simulink model "PIhigh"  (R2025a)
settings: Solver=VariableStepAuto  StartTime=0.0  StopTime=0.05  MaxStep=1e-9  RelTol=1e-3
libraries: spsVoltageMeasurementLib x5, spsSeriesRLCBranchLib x4, spsCurrentMeasurementLib x4, spsDiodeLib x2, spsMosfetLib x2, spsDCVoltageSourceLib x1, spsLinearTransformerLib x1, sps_lib x1
settings Model: Creator=FCH  LastModifiedBy=FCH
settings DataIOCC: ReturnWorkspaceOutputs=off

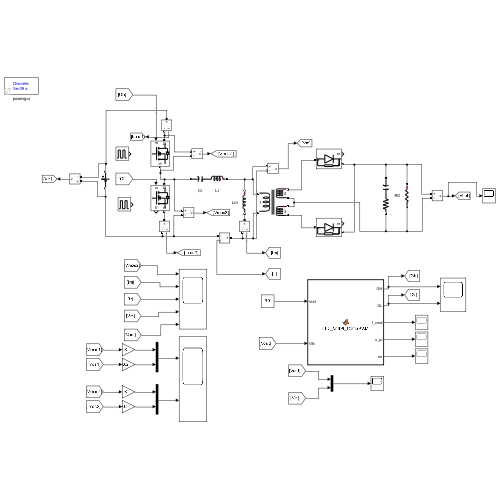
[thumbnail: Simulink's stored preview of the top-level diagram]
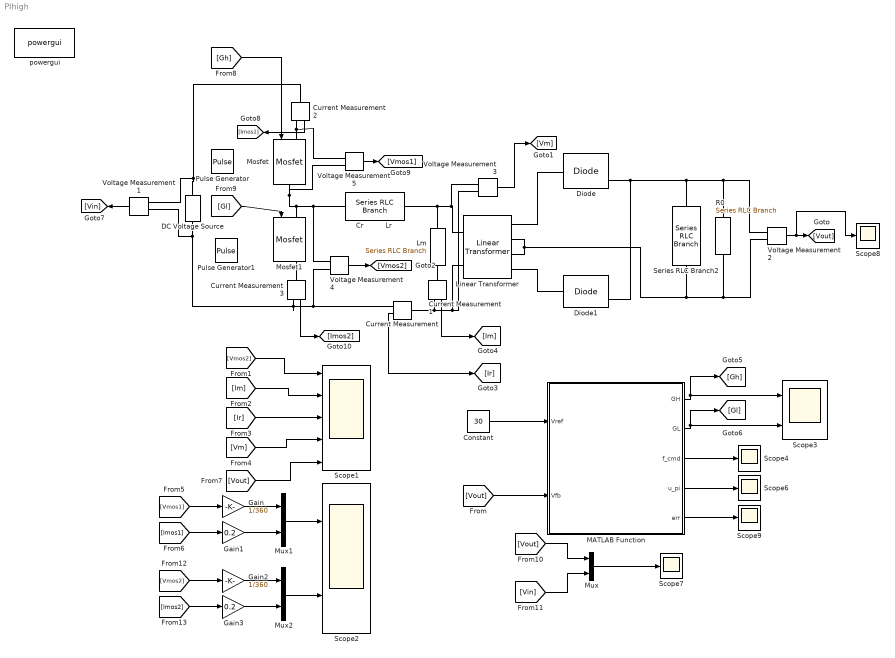
== system PIhigh ==
  Constant : Constant  Value=30
  Cr           Lr : spsSeriesRLCBranchLib/Series RLC Branch  LConnTagsString=__new0  RConnTagsString=__new0  BranchType=LC  Resistance=1  Inductance=18e-6  SetiL0=off  InitialCurrent=0  Capacitance=36e-9  Setx0=off  InitialVoltage=0  Measurements=None
  Current Measurement{,1..3} (4 alike) : spsCurrentMeasurementLib/Current Measurement  PhasorSimulation=off  OutputType=Complex  PSBequivalent=0
  DC Voltage Source : spsDCVoltageSourceLib/DC Voltage Source  Amplitude=400  Measurements=None
  Diode : spsDiodeLib/Diode  Ron=0.001  Lon=0  Vf=0.8  IC=0  UseSnubber=0  Rs=500  Cs=250e-9  Measurements=on
  Diode1 : spsDiodeLib/Diode  Ron=0.001  Lon=0  Vf=0.8  IC=0  UseSnubber=0  Rs=500  Cs=250e-9  Measurements=on
  Gain : Gain  Gain=1/360
  Gain1 : Gain  Gain=0.2
  Gain2 : Gain  Gain=1/360
  Gain3 : Gain  Gain=0.2
  Linear Transformer : spsLinearTransformerLib/Linear Transformer  UNITS=SI  NominalPower=[ 250e2 180e3 ]  winding1=[10 0 0]  winding2=[1 0 0]  ThreeWindings=on  winding3=[1 0 0]  RmLm=[inf inf]  Measurements=None  DataType=on
  Lm : spsSeriesRLCBranchLib/Series RLC Branch  LConnTagsString=__new0  RConnTagsString=__new0  BranchType=L  Resistance=1  Inductance=100e-6  SetiL0=off  InitialCurrent=0  Capacitance=1e-6  Setx0=off  InitialVoltage=0  Measurements=None
  MATLAB Function : MATLAB Function  TreatAsAtomicUnit=on
  Mosfet : spsMosfetLib/Mosfet  Ron=0.1  Lon=0  Rd=0.01  Vfd=0  IC=0  Rs=1e5  Cs=389e-1  Measurements=off
  Mosfet1 : spsMosfetLib/Mosfet  Ron=0.1  Lon=0  Rd=0.01  Vfd=0  IC=0  Rs=1e5  Cs=389e-12  Measurements=on
  Mux : Mux  Inputs=2
  Mux1 : Mux  Inputs=2
  Mux2 : Mux  Inputs=2
  Pulse Generator : DiscretePulseGenerator  PulseType=Time based  Period=1/270e2  PulseWidth=45
  Pulse Generator1 : DiscretePulseGenerator  PulseType=Time based  Period=1/270e2  PulseWidth=45  PhaseDelay=180/360*1/270e2
  R0 : spsSeriesRLCBranchLib/Series RLC Branch  LConnTagsString=__new0  RConnTagsString=__new0  BranchType=R  Resistance=10000  Inductance=1e-3  SetiL0=off  InitialCurrent=0  Capacitance=1e-6  Setx0=off  InitialVoltage=0  Measurements=Branch voltage
  Scope1 : Scope  NumInputPorts=5
      settings: ActiveDisplayYMinimum=-45.097156746790269  ActiveDisplayYMaximum=405.0968315999923
  Scope2 : Scope  NumInputPorts=2
      settings: ActiveDisplayYMinimum=-2.2545286858856493  ActiveDisplayYMaximum=1.9388480706148599
  Scope3 : Scope  NumInputPorts=2
      settings: ActiveDisplayYMinimum=-0.12499999999999997  ActiveDisplayYMaximum=1.125  DataLoggingVariableName=ScopeData3
  Scope{4,6..9} (5 alike) : Scope
      Scope4 settings: ActiveDisplayYMinimum=214374.4138129011  ActiveDisplayYMaximum=228140.57300499929  DataLoggingVariableName=ScopeData4
      Scope6 settings: ActiveDisplayYMinimum=-44.999999999999972  ActiveDisplayYMaximum=404.99999999999994  DataLoggingVariableName=ScopeData6
      Scope7 settings: ActiveDisplayYMinimum=-44.999999999999972  ActiveDisplayYMaximum=404.99999999999994  DataLoggingVariableName=ScopeData2
      Scope8 settings: ActiveDisplayYMinimum=-6.1893685032288337  ActiveDisplayYMaximum=55.704316529059234  DataLoggingVariableName=U_output
      Scope9 settings: ActiveDisplayYMinimum=-25.704316529059234  ActiveDisplayYMaximum=36.189368503228835  DataLoggingVariableName=ScopeData8
  Series RLC Branch2 : spsSeriesRLCBranchLib/Series RLC Branch  LConnTagsString=__new0  RConnTagsString=__new0  BranchType=RC  Resistance=0.01  Inductance=1e-3  SetiL0=off  InitialCurrent=0  Capacitance=1e-6  Setx0=off  InitialVoltage=0  Measurements=None
  Voltage Measurement{1..5} (5 alike) : spsVoltageMeasurementLib/Voltage Measurement  PhasorSimulation=off  OutputType=Complex  PSBequivalent=0
  powergui : sps_lib/powergui  Priority=1  SimulationMode=Discrete  SampleTime=1/(200e6)  frequency=60  Iterations=50  frequencyindice=0  Pbase=100e6  ErrMax=1e-4  UnitsV=kV  UnitsW=MW  buscounter=0  FunctionMessages=off  echomessages=off  EnableUseOfTLC=off  CurrentSourceSwitches=off  DisableSnubberDevices=off  DisableRonSwitches=off  DisableVfSwitches=off  DisplayEquations=off  AutomaticDiscreteSolvers=off  SolverType=Tustin/Backward Euler (TBE)  Interpol=off  ExternalGateDelay=off  methode=off  Ts=100  x0status=blocks  SPID=on  SwTol=0  HookPort=off  NonlinearTolerance=1e-4  nMaxIteration=100  ContinueOnMaxIteration=off  RestoreLinks=warning  ResistiveCurrentMeasurement=off  Frange=[0:2:500]  Ylog=off  Xlog=on  ShowGrid=off  save=off  variable=ZData  structure=0  ZoomFFT=off  StartTime=0.0  cycles=1  DisplayStyle=1  fundamental=60  FreqAxis=off  MaxFrequency=1000  frequencyindicesteady=1  RmsSteady=1  display=off
  wires:
  Voltage Measurement2/1 -> Scope8/1, [Vout]
  Constant/1 -> MATLAB Function/1(Vref)
  [Vout] -> MATLAB Function/2(Vfb)
  MATLAB Function/1(GH) -> [Gh], Scope3/1
  MATLAB Function/2(GL) -> [Gl], Scope3/2
  MATLAB Function/4(u_pi) -> Scope6/1
  MATLAB Function/3(f_cmd) -> Scope4/1
  MATLAB Function/5(err) -> Scope9/1
  Voltage Measurement3/1 -> [Vm]
  Voltage Measurement4/1 -> [Vmos2]
  Current Measurement/1 -> [Ir]
  Current Measurement1/1 -> [Im]
  [Vmos2] -> Scope1/1
  [Im] -> Scope1/2
  [Ir] -> Scope1/3
  [Vm] -> Scope1/4
  [Vout] -> Scope1/5
  Mux/1 -> Scope7/1
  [Vout] -> Mux/1
  Voltage Measurement1/1 -> [Vin]
  [Vin] -> Mux/2
  [Gl] -> Mosfet1/1
  [Gh] -> Mosfet/1
  Current Measurement2/1 -> [Imos1]
  Voltage Measurement5/1 -> [Vmos1]
  Current Measurement3/1 -> [Imos2]
  [Vmos1] -> Gain/1
  [Imos1] -> Gain1/1
  Mux1/1 -> Scope2/1
  [Vmos2] -> Gain2/1
  [Imos2] -> Gain3/1
  Mux2/1 -> Scope2/2
  Gain/1 -> Mux1/1
  Gain1/1 -> Mux1/2
  Gain2/1 -> Mux2/1
  Gain3/1 -> Mux2/2
  connections:
  DC Voltage Source/RConn1 -- Voltage Measurement1/LConn2 -- Current Measurement2/LConn1
  Mosfet/RConn1 -- Voltage Measurement4/LConn1 -- Cr           Lr/RConn1 -- Mosfet1/LConn1 -- Voltage Measurement5/LConn2
  Lm/RConn1 -- Current Measurement1/LConn1
  Cr           Lr/LConn1 -- Voltage Measurement3/LConn1 -- Linear Transformer/LConn1 -- Lm/LConn1
  Linear Transformer/RConn1 -- Diode/LConn1
  Diode/RConn1 -- Diode1/RConn1 -- Series RLC Branch2/RConn1 -- R0/LConn1 -- Voltage Measurement2/LConn1
  R0/RConn1 -- Voltage Measurement2/LConn2 -- Linear Transformer/RConn2 -- Linear Transformer/RConn3 -- Series RLC Branch2/LConn1
  Linear Transformer/RConn4 -- Diode1/LConn1
  Current Measurement/RConn1 -- Voltage Measurement1/LConn1 -- DC Voltage Source/LConn1 -- Current Measurement3/RConn1 -- Voltage Measurement4/LConn2
  Linear Transformer/LConn2 -- Voltage Measurement3/LConn2 -- Current Measurement1/RConn1 -- Current Measurement/LConn1
  Current Measurement2/RConn1 -- Voltage Measurement5/LConn1 -- Mosfet/LConn1
  Mosfet1/RConn1 -- Current Measurement3/LConn1

== matlab function PIhigh/MATLAB Function ==
  data: Vref input; GH output; Vfb input; GL output; f_cmd output; u_pi output; err output
 function [GH, GL, f_cmd, u_pi,err] = LLC_VoltPI_CompPWM(Vref, Vfb)
%#codegen
% LLC 变换器 PI 电压闭环 + 互补 PWM 驱动（变频控制）
% 输入:
%   Vref  - 输出电压给定 (V)
%   Vfb   - 输出电压反馈 (V)
% 输出:
%   GH    - 高桥臂驱动（逻辑 0/1）
%   GL    - 低桥臂驱动（逻辑 0/1），与 GH 互补且带死区
%   f_cmd - 当前开关频率命令 (Hz)，便于观察
%   u_pi  - PI 控制器输出（归一化调节量，便于调试）

%% ========= 用户根据实际系统需要修改的参数 =========

% --- 控制周期（与 MATLAB Function 调用步长一致） ---
% Ts = 1/(270e3*20);          % 1 us 控制周期，例如 MCU 1 MHz ISR
Ts = 1/(2000e6);          % 1 us 控制周期，例如 MCU 1 MHz ISR
% --- PI 参数（电压环）---
Kp = 0.00001;           % 比例系数
Ki = 50;            % 积分系数

% --- LLC 开关频率范围 ---
f_min = 180e3;       % 最低频率 (Hz)
f_max = 270e3;      % 最高频率 (Hz)

% --- 死区时间 ---
t_dead = 200e-9;    % 2 ns 死区，根据驱动/器件调整

% --- 积分项限幅，防止积分饱和 ---
ui_max = 0.5;
ui_min = -0.5;

%% ========= 持久变量（只初始化一次） =========
persistent ui t_half leg dead_t
if isempty(ui)
    ui      = 0;        % PI 积分项
    t_half  = 0;        % 半周期计时
    leg     = int8(0);  % 当前导通臂：0=上臂导通，1=下臂导通
    dead_t  = 0;        % 当前死区计时
end

%% ========= 1. 电压误差 & PI 电压环 =========
err = Vref - Vfb;      % 电压误差：Vref - Vfb

% 比例项
up = Kp * err;

% 积分项更新
ui = ui + Ki * Ts * err;

% 积分限幅
if ui > ui_max
    ui = ui_max;
elseif ui < ui_min
    ui = ui_min;
end

% PI 输出
u_pi = up + ui;

%% ========= 2. PI 输出映射为开关频率命令 =========
% 假设 u_pi 在 [-1, 1] 范围内有效，这里再做一次限幅
if u_pi > 1
    u_pi = 1;
elseif u_pi < -1
    u_pi = -1;
end

% u_pi [-1,1] -> u_norm [0,1]
u_norm = 0.5 + 0.5 * u_pi;

% 再保证在 [0,1] 内
if u_norm > 1
    u_norm = 1;
elseif u_norm < 0
    u_norm = 0;
end

% 映射到频率范围 [f_min, f_max]
f_cmd = f_min + u_norm * (f_max - f_min);

% 保险再限幅
if f_cmd > f_max
    f_cmd = f_max;
elseif f_cmd < f_min
    f_cmd = f_min;
end

%% ========= 3. 根据频率命令生成 50% 占空方波 =========
% 半周期 = 1 / (2 * f_cmd)
T_half = 1.0 / (2.0 * f_cmd);

% 半周期计数
t_half = t_half + Ts;

% 每经过一个半周期翻转一次桥臂导通状态
if t_half >= T_half
    t_half = t_half - T_half;     % 保持时间误差不积累
    leg    = bitxor(leg, int8(1));% 0 <-> 1 翻转导通臂
    dead_t = t_dead;              % 每次换向都重新启动死区
end

%% ========= 4. 互补 PWM + 死区逻辑 =========
% 在死区时间内，两臂都关闭
if dead_t > 0
    dead_t = dead_t - Ts;
    GH = false;
    GL = false;
else
    % 死区结束后，根据 leg 状态驱动互补 PWM
    if leg == 0
        GH = true;     % 上臂导通
        GL = false;    % 下臂关闭
    else
        GH = false;    % 上臂关闭
        GL = true;     % 下臂导通
    end
end

end
